simulink model "Reducing_the_Harmonics_Impact_H2"  (R2023b)
settings: Solver=ode1  StartTime=0.0  StopTime=0.2  FixedStep=1e-6  RelTol=1e-3
libraries: spsSeriesRLCBranchLib x28, spsGroundLib x7, spsCurrentMeasurementLib x4, spsACVoltageSourceLib x3, eeGeneralControl x3, dspstat3 x2, spsTHDLib x2, spsVoltageMeasurementLib x2, spsUniversalBridgeLib x1, sps_lib x1
settings Model: Creator=ASUS  LastModifiedBy=ASUS
settings DataIOCC: ReturnWorkspaceOutputs=off

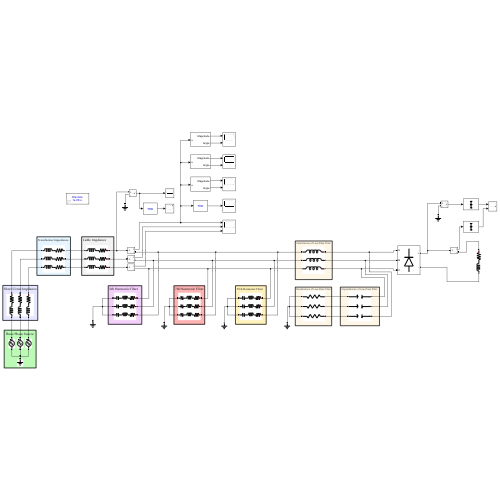
[thumbnail: Simulink's stored preview of the top-level diagram]
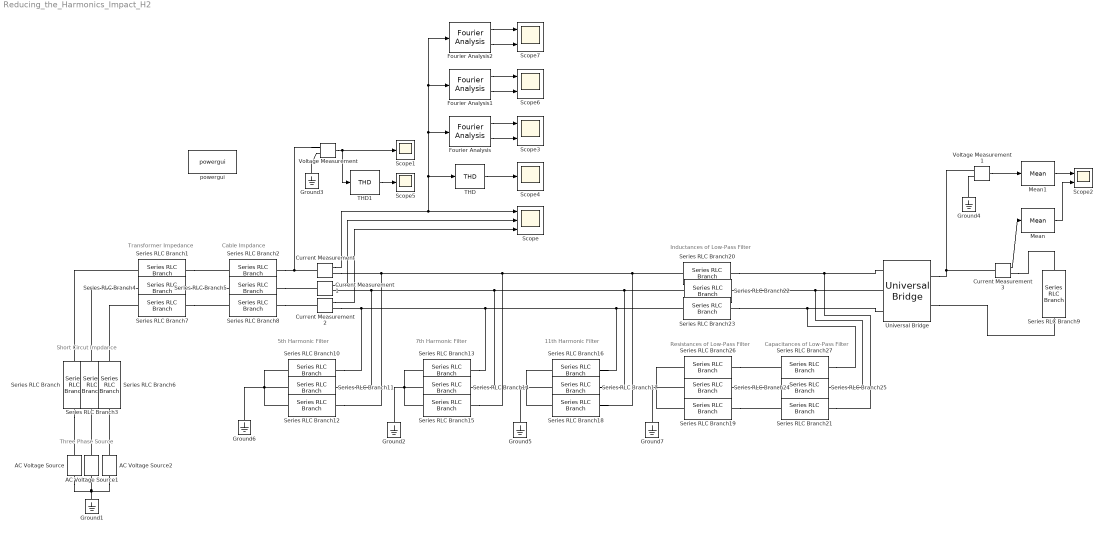
== system Reducing_the_Harmonics_Impact_H2 ==
  note: Inductances of Low-Pass Filter
  note: Capacitances of Low-Pass Filter
  note: Resistances of Low-Pass Filter
  note: 11th Harmonic Filter
  note: 7th Harmonic Filter
  note: 5th Harmonic Filter
  note: Cable Impdance
  note: Transformer Impedance
  note: Three Phase Source
  note: Short Circut Impdance
  AC Voltage Source : spsACVoltageSourceLib/AC Voltage Source  Amplitude=220*sqrt(2)  Phase=0  Frequency=50  SampleTime=0  Measurements=None  BusType=swing  Pref=10e3  Qref=0  Qmin=-inf  Qmax=+inf
  AC Voltage Source1 : spsACVoltageSourceLib/AC Voltage Source  Amplitude=220*sqrt(2)  Phase=120  Frequency=50  SampleTime=0  Measurements=None  BusType=swing  Pref=10e3  Qref=0  Qmin=-inf  Qmax=+inf
  AC Voltage Source2 : spsACVoltageSourceLib/AC Voltage Source  Amplitude=220*sqrt(2)  Phase=240  Frequency=50  SampleTime=0  Measurements=None  BusType=swing  Pref=10e3  Qref=0  Qmin=-inf  Qmax=+inf
  Current Measurement{,1..3} (4 alike) : spsCurrentMeasurementLib/Current Measurement  PhasorSimulation=off  OutputType=Complex  PSBequivalent=0
  Fourier Analysis : eeGeneralControl/Fourier Analysis  f=50  n=5  M0=0  Ph0=0  BufferSize=8192  Ts=-1
      settings: LibrarySourceBlock=ee_sl_lib/General Control/Fourier Analysis
  Fourier Analysis1 : eeGeneralControl/Fourier Analysis  f=50  n=7  M0=0  Ph0=0  BufferSize=8192  Ts=-1
      settings: LibrarySourceBlock=ee_sl_lib/General Control/Fourier Analysis
  Fourier Analysis2 : eeGeneralControl/Fourier Analysis  f=50  n=11  M0=0  Ph0=0  BufferSize=8192  Ts=-1
      settings: LibrarySourceBlock=ee_sl_lib/General Control/Fourier Analysis
  Ground{1..7} (7 alike) : spsGroundLib/Ground  LConnTagsString=a
  Mean : dspstat3/Mean  run=off  InputProcessing=Columns as channels (frame based)  reset_popup=None  directionMode=Each column  dimension=1  roiEnable=off  roiType=Rectangles  roiPortion=Entire ROI  roiOutput=Individual statistics for each ROI  roiFlag=off  roundingMode=Floor  overflowMode=off  outputDataTypeStr=Inherit: Same as accumulator  outputMin=[]  outputMax=[]  outputLastDataTypeStr=Inherit: Same as accumulator
  Mean1 : dspstat3/Mean  run=off  InputProcessing=Columns as channels (frame based)  reset_popup=None  directionMode=Each column  dimension=1  roiEnable=off  roiType=Rectangles  roiPortion=Entire ROI  roiOutput=Individual statistics for each ROI  roiFlag=off  roundingMode=Floor  overflowMode=off  outputDataTypeStr=Inherit: Same as accumulator  outputMin=[]  outputMax=[]  outputLastDataTypeStr=Inherit: Same as accumulator
  Scope : Scope  NumInputPorts=3
  Scope1 : Scope
  Scope{2..3,6..7} (4 alike) : Scope  NumInputPorts=2
  Scope4 : Scope
  Scope5 : Scope
  Series RLC Branch : spsSeriesRLCBranchLib/Series RLC Branch  LConnTagsString=__new0  RConnTagsString=__new0  BranchType=RL  Resistance=3.184e-3  Inductance=1e-3  SetiL0=off  InitialCurrent=0  Capacitance=1e-6  Setx0=off  InitialVoltage=0  Measurements=None
  Series RLC Branch1 : spsSeriesRLCBranchLib/Series RLC Branch  LConnTagsString=__new0  RConnTagsString=__new0  BranchType=RL  Resistance=2.08e-3  Inductance=9.6e-3/314  SetiL0=off  InitialCurrent=0  Capacitance=1e-6  Setx0=off  InitialVoltage=0  Measurements=None
  Series RLC Branch10 : spsSeriesRLCBranchLib/Series RLC Branch  LConnTagsString=__new0  RConnTagsString=__new0  BranchType=RLC  Resistance=0.253  Inductance=0.0121  SetiL0=off  InitialCurrent=0  Capacitance=3.339e-5  Setx0=off  InitialVoltage=0  Measurements=None
  Series RLC Branch11 : spsSeriesRLCBranchLib/Series RLC Branch  LConnTagsString=__new0  RConnTagsString=__new0  BranchType=RLC  Resistance=0.253  Inductance=0.0121  SetiL0=off  InitialCurrent=0  Capacitance=3.339e-5  Setx0=off  InitialVoltage=0  Measurements=None
  Series RLC Branch12 : spsSeriesRLCBranchLib/Series RLC Branch  LConnTagsString=__new0  RConnTagsString=__new0  BranchType=RLC  Resistance=0.253  Inductance=0.0121  SetiL0=off  InitialCurrent=0  Capacitance=3.339e-5  Setx0=off  InitialVoltage=0  Measurements=None
  Series RLC Branch13 : spsSeriesRLCBranchLib/Series RLC Branch  LConnTagsString=__new0  RConnTagsString=__new0  BranchType=RLC  Resistance=0.1815  Inductance=0.00619  SetiL0=off  InitialCurrent=0  Capacitance=3.339e-5  Setx0=off  InitialVoltage=0  Measurements=None
  Series RLC Branch14 : spsSeriesRLCBranchLib/Series RLC Branch  LConnTagsString=__new0  RConnTagsString=__new0  BranchType=RLC  Resistance=0.1815  Inductance=0.00619  SetiL0=off  InitialCurrent=0  Capacitance=3.339e-5  Setx0=off  InitialVoltage=0  Measurements=None
  Series RLC Branch15 : spsSeriesRLCBranchLib/Series RLC Branch  LConnTagsString=__new0  RConnTagsString=__new0  BranchType=RLC  Resistance=0.1815  Inductance=0.00619  SetiL0=off  InitialCurrent=0  Capacitance=3.339e-5  Setx0=off  InitialVoltage=0  Measurements=None
  Series RLC Branch16 : spsSeriesRLCBranchLib/Series RLC Branch  LConnTagsString=__new0  RConnTagsString=__new0  BranchType=RLC  Resistance=0.115  Inductance=0.0025  SetiL0=off  InitialCurrent=0  Capacitance=3.339e-5  Setx0=off  InitialVoltage=0  Measurements=None
  Series RLC Branch17 : spsSeriesRLCBranchLib/Series RLC Branch  LConnTagsString=__new0  RConnTagsString=__new0  BranchType=RLC  Resistance=0.115  Inductance=0.0025  SetiL0=off  InitialCurrent=0  Capacitance=3.339e-5  Setx0=off  InitialVoltage=0  Measurements=None
  Series RLC Branch18 : spsSeriesRLCBranchLib/Series RLC Branch  LConnTagsString=__new0  RConnTagsString=__new0  BranchType=RLC  Resistance=0.115  Inductance=0.0025  SetiL0=off  InitialCurrent=0  Capacitance=3.339e-5  Setx0=off  InitialVoltage=0  Measurements=None
  Series RLC Branch19 : spsSeriesRLCBranchLib/Series RLC Branch  LConnTagsString=__new0  RConnTagsString=__new0  BranchType=R  Resistance=0.628  Inductance=0.0025  SetiL0=off  InitialCurrent=0  Capacitance=3.339e-5  Setx0=off  InitialVoltage=0  Measurements=None
  Series RLC Branch2 : spsSeriesRLCBranchLib/Series RLC Branch  LConnTagsString=__new0  RConnTagsString=__new0  BranchType=RL  Resistance=0.256  Inductance=6.05e-5  SetiL0=off  InitialCurrent=0  Capacitance=1e-6  Setx0=off  InitialVoltage=0  Measurements=None
  Series RLC Branch20 : spsSeriesRLCBranchLib/Series RLC Branch  LConnTagsString=__new0  RConnTagsString=__new0  BranchType=L  Resistance=0.115  Inductance=0.002  SetiL0=off  InitialCurrent=0  Capacitance=3.339e-5  Setx0=off  InitialVoltage=0  Measurements=None
  Series RLC Branch21 : spsSeriesRLCBranchLib/Series RLC Branch  LConnTagsString=__new0  RConnTagsString=__new0  BranchType=C  Resistance=0.115  Inductance=0.0025  SetiL0=off  InitialCurrent=0  Capacitance=562.9e-6  Setx0=off  InitialVoltage=0  Measurements=None
  Series RLC Branch22 : spsSeriesRLCBranchLib/Series RLC Branch  LConnTagsString=__new0  RConnTagsString=__new0  BranchType=L  Resistance=0.115  Inductance=0.002  SetiL0=off  InitialCurrent=0  Capacitance=3.339e-5  Setx0=off  InitialVoltage=0  Measurements=None
  Series RLC Branch23 : spsSeriesRLCBranchLib/Series RLC Branch  LConnTagsString=__new0  RConnTagsString=__new0  BranchType=L  Resistance=0.115  Inductance=0.002  SetiL0=off  InitialCurrent=0  Capacitance=3.339e-5  Setx0=off  InitialVoltage=0  Measurements=None
  Series RLC Branch24 : spsSeriesRLCBranchLib/Series RLC Branch  LConnTagsString=__new0  RConnTagsString=__new0  BranchType=R  Resistance=0.628  Inductance=0.0025  SetiL0=off  InitialCurrent=0  Capacitance=3.339e-5  Setx0=off  InitialVoltage=0  Measurements=None
  Series RLC Branch25 : spsSeriesRLCBranchLib/Series RLC Branch  LConnTagsString=__new0  RConnTagsString=__new0  BranchType=C  Resistance=0.115  Inductance=0.0025  SetiL0=off  InitialCurrent=0  Capacitance=562.9e-6  Setx0=off  InitialVoltage=0  Measurements=None
  Series RLC Branch26 : spsSeriesRLCBranchLib/Series RLC Branch  LConnTagsString=__new0  RConnTagsString=__new0  BranchType=R  Resistance=0.628  Inductance=0.0025  SetiL0=off  InitialCurrent=0  Capacitance=3.339e-5  Setx0=off  InitialVoltage=0  Measurements=None
  Series RLC Branch27 : spsSeriesRLCBranchLib/Series RLC Branch  LConnTagsString=__new0  RConnTagsString=__new0  BranchType=C  Resistance=0.115  Inductance=0.0025  SetiL0=off  InitialCurrent=0  Capacitance=562.9e-6  Setx0=off  InitialVoltage=0  Measurements=None
  Series RLC Branch3 : spsSeriesRLCBranchLib/Series RLC Branch  LConnTagsString=__new0  RConnTagsString=__new0  BranchType=RL  Resistance=3.184e-3  Inductance=1e-3  SetiL0=off  InitialCurrent=0  Capacitance=1e-6  Setx0=off  InitialVoltage=0  Measurements=None
  Series RLC Branch4 : spsSeriesRLCBranchLib/Series RLC Branch  LConnTagsString=__new0  RConnTagsString=__new0  BranchType=RL  Resistance=2.08e-3  Inductance=9.6e-3/314  SetiL0=off  InitialCurrent=0  Capacitance=1e-6  Setx0=off  InitialVoltage=0  Measurements=None
  Series RLC Branch5 : spsSeriesRLCBranchLib/Series RLC Branch  LConnTagsString=__new0  RConnTagsString=__new0  BranchType=RL  Resistance=0.256  Inductance=6.05e-5  SetiL0=off  InitialCurrent=0  Capacitance=1e-6  Setx0=off  InitialVoltage=0  Measurements=None
  Series RLC Branch6 : spsSeriesRLCBranchLib/Series RLC Branch  LConnTagsString=__new0  RConnTagsString=__new0  BranchType=RL  Resistance=3.184e-3  Inductance=1e-3  SetiL0=off  InitialCurrent=0  Capacitance=1e-6  Setx0=off  InitialVoltage=0  Measurements=None
  Series RLC Branch7 : spsSeriesRLCBranchLib/Series RLC Branch  LConnTagsString=__new0  RConnTagsString=__new0  BranchType=RL  Resistance=2.08e-3  Inductance=9.6e-3/314  SetiL0=off  InitialCurrent=0  Capacitance=1e-6  Setx0=off  InitialVoltage=0  Measurements=None
  Series RLC Branch8 : spsSeriesRLCBranchLib/Series RLC Branch  LConnTagsString=__new0  RConnTagsString=__new0  BranchType=RL  Resistance=0.256  Inductance=6.05e-5  SetiL0=off  InitialCurrent=0  Capacitance=1e-6  Setx0=off  InitialVoltage=0  Measurements=None
  Series RLC Branch9 : spsSeriesRLCBranchLib/Series RLC Branch  LConnTagsString=__new0  RConnTagsString=__new0  BranchType=RL  Resistance=10.6  Inductance=1e-4  SetiL0=off  InitialCurrent=0  Capacitance=1e-6  Setx0=off  InitialVoltage=0  Measurements=None
  THD : spsTHDLib/THD  Freq=50  Ts=0
  THD1 : spsTHDLib/THD  Freq=50  Ts=0
  Universal Bridge : spsUniversalBridgeLib/Universal Bridge  Arms=3  SnubberResistance=2000  SnubberCapacitance=50e-9  Device=Diodes  Ron=0.01  Lon=0  ForwardVoltages="[  0  0  ]"  ForwardVoltage=0.8  GTOparameters=[ 10e-6 , 20e-6 ]  IGBTparameters=[ 1e-6 , 2e-6 ]  Measurements=None  Measurements_2=None  converterType=Rectifier
  Voltage Measurement : spsVoltageMeasurementLib/Voltage Measurement  PhasorSimulation=off  OutputType=Complex  PSBequivalent=0
  Voltage Measurement1 : spsVoltageMeasurementLib/Voltage Measurement  PhasorSimulation=off  OutputType=Complex  PSBequivalent=0
  powergui : sps_lib/powergui  Priority=1  SimulationMode=Discrete  SampleTime=1e-6  frequency=60  Iterations=50  frequencyindice=50  Pbase=100e6  ErrMax=1e-4  UnitsV=kV  UnitsW=MW  buscounter=0  FunctionMessages=off  echomessages=off  EnableUseOfTLC=off  CurrentSourceSwitches=off  DisableSnubberDevices=off  DisableRonSwitches=off  DisableVfSwitches=off  DisplayEquations=off  AutomaticDiscreteSolvers=off  SolverType=Tustin/Backward Euler (TBE)  Interpol=off  ExternalGateDelay=off  methode=off  Ts=100  x0status=blocks  SPID=on  SwTol=0  HookPort=off  NonlinearTolerance=1e-4  nMaxIteration=100  ContinueOnMaxIteration=off  RestoreLinks=warning  ResistiveCurrentMeasurement=off  Frange=[0:2:500]  Ylog=off  Xlog=on  ShowGrid=off  save=off  variable=ZData  structure=0  ZoomFFT=off  StartTime=0.0  cycles=1  DisplayStyle=1  fundamental=60  FreqAxis=off  MaxFrequency=1000  frequencyindicesteady=1  RmsSteady=1  display=off
  wires:
  Current Measurement/1 -> THD/1, Fourier Analysis/1, Fourier Analysis1/1, Fourier Analysis2/1, Scope/1
  Current Measurement1/1 -> Scope/2
  Current Measurement2/1 -> Scope/3
  Voltage Measurement/1 -> THD1/1, Scope1/1
  Current Measurement3/1 -> Mean/1
  Mean/1 -> Scope2/2
  Voltage Measurement1/1 -> Mean1/1
  Mean1/1 -> Scope2/1
  THD/1 -> Scope4/1
  THD1/1 -> Scope5/1
  Fourier Analysis/1 -> Scope3/1
  Fourier Analysis/2 -> Scope3/2
  Fourier Analysis1/1 -> Scope6/1
  Fourier Analysis2/1 -> Scope7/1
  Fourier Analysis2/2 -> Scope7/2
  Fourier Analysis1/2 -> Scope6/2
  connections:
  Ground1/LConn1 -- AC Voltage Source/LConn1 -- AC Voltage Source2/LConn1 -- AC Voltage Source1/LConn1
  Series RLC Branch/RConn1 -- AC Voltage Source/RConn1
  Series RLC Branch1/RConn1 -- Series RLC Branch/LConn1
  Series RLC Branch1/LConn1 -- Series RLC Branch2/RConn1
  Series RLC Branch4/LConn1 -- Series RLC Branch5/RConn1
  Series RLC Branch4/RConn1 -- Series RLC Branch3/LConn1
  Series RLC Branch7/RConn1 -- Series RLC Branch6/LConn1
  Series RLC Branch7/LConn1 -- Series RLC Branch8/RConn1
  AC Voltage Source2/RConn1 -- Series RLC Branch6/RConn1
  AC Voltage Source1/RConn1 -- Series RLC Branch3/RConn1
  Series RLC Branch8/LConn1 -- Current Measurement2/LConn1
  Series RLC Branch5/LConn1 -- Current Measurement1/LConn1
  Series RLC Branch2/LConn1 -- Voltage Measurement/LConn1 -- Current Measurement/LConn1
  Series RLC Branch22/RConn1 -- Series RLC Branch17/LConn1 -- Series RLC Branch14/LConn1 -- Series RLC Branch11/LConn1 -- Current Measurement1/RConn1
  Current Measurement2/RConn1 -- Series RLC Branch10/LConn1 -- Series RLC Branch16/LConn1 -- Series RLC Branch23/RConn1 -- Series RLC Branch13/LConn1
  Current Measurement/RConn1 -- Series RLC Branch18/LConn1 -- Series RLC Branch20/RConn1 -- Series RLC Branch15/LConn1 -- Series RLC Branch12/LConn1
  Ground3/LConn1 -- Voltage Measurement/LConn2
  Universal Bridge/RConn2 -- Series RLC Branch9/RConn1
  Ground4/LConn1 -- Voltage Measurement1/LConn2
  Ground6/LConn1 -- Series RLC Branch12/RConn1 -- Series RLC Branch10/RConn1 -- Series RLC Branch11/RConn1
  Series RLC Branch13/RConn1 -- Series RLC Branch15/RConn1 -- Ground2/LConn1 -- Series RLC Branch14/RConn1
  Ground5/LConn1 -- Series RLC Branch16/RConn1 -- Series RLC Branch18/RConn1 -- Series RLC Branch17/RConn1
  Universal Bridge/RConn1 -- Voltage Measurement1/LConn1 -- Current Measurement3/LConn1
  Current Measurement3/RConn1 -- Series RLC Branch9/LConn1
  Series RLC Branch20/LConn1 -- Series RLC Branch21/LConn1 -- Universal Bridge/LConn1
  Universal Bridge/LConn2 -- Series RLC Branch22/LConn1 -- Series RLC Branch25/LConn1
  Series RLC Branch23/LConn1 -- Series RLC Branch27/LConn1 -- Universal Bridge/LConn3
  Series RLC Branch19/LConn1 -- Series RLC Branch21/RConn1
  Series RLC Branch24/LConn1 -- Series RLC Branch25/RConn1
  Series RLC Branch26/LConn1 -- Series RLC Branch27/RConn1
  Series RLC Branch19/RConn1 -- Series RLC Branch24/RConn1 -- Ground7/LConn1 -- Series RLC Branch26/RConn1
